simulink model "MZ_Simulink_AAI"  (R2020a)
settings: Solver=FixedStepAuto  StartTime=0.0  StopTime=10.0  FixedStep=1e-3  RelTol=1e-3  EnableMultiTasking=on
undefined symbols (not defined in the file or in its folder): D0, D1, D10, D11, D12, D13, D2, D3, D5, D6, D8, D9, Modes, PTA0, PTA1, PTA2, PTB9, PTC16, PTC17, PTC2, PTC4, PTD0, PTD1, PTD2, PTD3
libraries: frdmk64flib x12, simulink x1
settings Model: ExtModeTrigDuration=5  Creator=USER  LastModifiedBy=micha
settings OptimizationCC: EnhancedBackFolding=on  PassReuseOutputArgsAs=Individual arguments  ZeroExternalMemoryAtStartup=off  ZeroInternalMemoryAtStartup=off  MaxStackSize=64  OptimizeBlockOrder=speed  DifferentSizesBufferReuse=on  OptimizationCustomize=off  EfficientTunableParamExpr=on
settings DebuggingCC: ParameterTunabilityLossMsg=error
settings HardwareCC: ProdBitPerPointer=32  ProdBitPerSizeT=32  ProdBitPerPtrDiffT=32  ProdLargestAtomicInteger=Long  ProdLargestAtomicFloat=Double  ProdWordSize=32  ProdHWDeviceType=ARM Compatible->ARM Cortex
settings SFSimCC: MATLABDynamicMemAlloc=off
settings RTWCC: SystemTargetFile=ert.tlc  HardwareBoard=NXP FRDM-K64F  TemplateMakefile=ert_default_tmf  Toolchain=GNU Tools for ARM Embedded Processors
settings CodeAppCC: ForceParamTrailComments=on  IgnoreCustomStorageClasses=off  OperatorAnnotations=on  SimulinkDataObjDesc=on  SFDataObjDesc=on  InsertBlockDesc=on

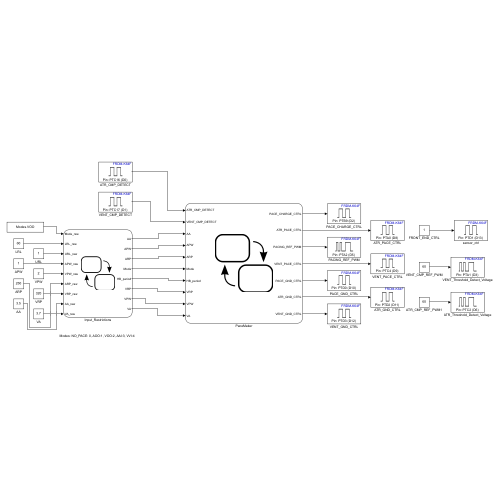
[thumbnail: Simulink's stored preview of the top-level diagram]
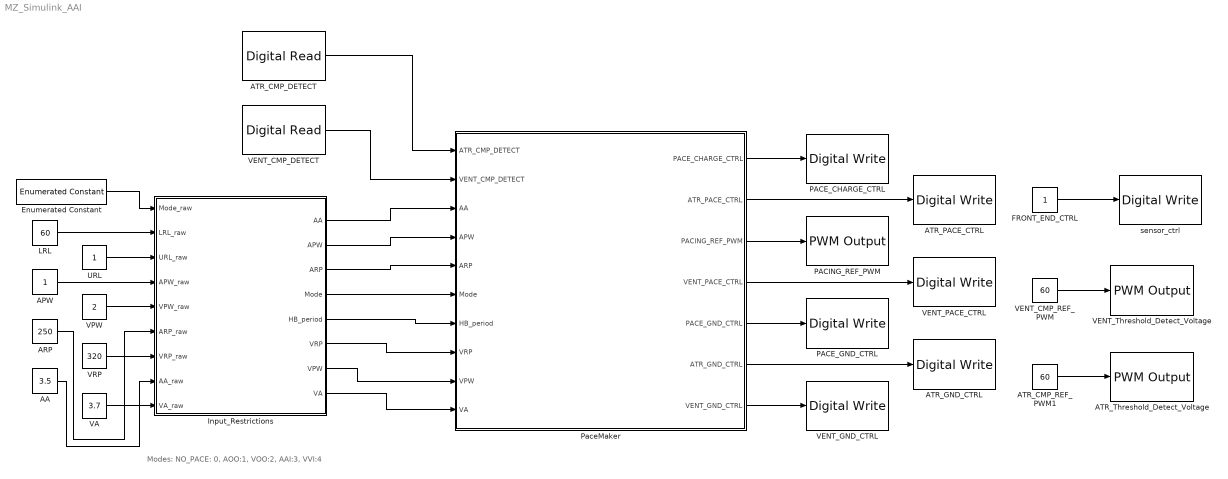
== system MZ_Simulink_AAI ==
  note: Modes: NO_PACE: 0, AOO:1, VOO:2, AAI:3, VVI:4
  AA : Constant  Value=3.5  OutDataTypeStr=single
  APW : Constant  OutDataTypeStr=uint8
  ARP : Constant  Value=250  OutDataTypeStr=uint16
  ATR_CMP_DETECT : frdmk64flib/Digital Read  Whichpin=PTC16 (D0)  SampleTime=-1
  ATR_CMP_REF_PWM1 : Constant  Value=60  OutDataTypeStr=uint8
  ATR_GND_CTRL : frdmk64flib/Digital Write  Whichpin=PTD2 (D11)
  ATR_PACE_CTRL : frdmk64flib/Digital Write  Whichpin=PTA0 (D8)
  ATR_Threshold_Detect_Voltage : frdmk64flib/PWM Output  Whichpin=PTC2 (D6)  InitialFrequency=2000  InitialDutyCycle=0
  Enumerated Constant : simulink/Sources/Enumerated Constant  OutDataTypeStr=Enum: Modes  Value=Modes.VOO  SampleTime=inf
  FRONT_END_CTRL : Constant
  Input_Restrictions : Stateflow chart  TreatAsAtomicUnit=on
      settings: PortSchema="{\"entries\":[{\"content\":{\"sides\":[{\"content\":{\"connectorIds\":[\"In1\",\"In2\",\"In3\",\"In4\",\"In5\",\"In6\",\"In7\",\"In8\",\"In9\"]},\"type\":\"ConnectorPlacement.EquallySpacedRectSide\",\"uuid\":\"6ca4b211-7758-4da9-b575-bca72ef3bde0\"},{\"content\":{\"connectorIds\":[\"Out6\",\"Out2\",\"Out4\",\"Out1\",\"Out8\",\"Out5\",\"Out3\",\"Out7\"],\"side\":\"RIGHT\"},\"type\":\"ConnectorPlacement.EquallySpacedRectSide\",\"uuid\":\"378f9a2c-b26e-4d35-a148-104ac3e5eb3b\"},{\"content\":{\"connectorIds\":[],\"side\":\"TOP\"},\"type\":\"ConnectorPlacement.EquallySpacedRectSide\",\"uuid\":\"60b5eb54-812a-46fe-8169-2e41f06633e9\"}]},\"type\":\"ConnectorPlacement.EquallySpacedConnector\",\"uuid\":\"c7c5acee-7732-4c88-8beb-9d710d5b10aa\"}],\"packageUris\":[\"http://schema.mathworks.com/mf0/Connector/R2020b\"],\"version\":\"1.0\"}"
  LRL : Constant  Value=60  OutDataTypeStr=uint8
  PACE_CHARGE_CTRL : frdmk64flib/Digital Write  Whichpin=PTB9 (D2)
  PACE_GND_CTRL : frdmk64flib/Digital Write  Whichpin=PTD0 (D10)
  PACING_REF_PWM : frdmk64flib/PWM Output  Whichpin=PTA2 (D5)  InitialFrequency=2000  InitialDutyCycle=0
  PaceMaker : Stateflow chart  TreatAsAtomicUnit=on
      settings: PortSchema="{\"entries\":[{\"content\":{\"sides\":[{\"content\":{\"connectorIds\":[\"In2\",\"In3\",\"In6\",\"In8\",\"In4\",\"In1\",\"In10\",\"In5\",\"In9\",\"In7\"]},\"type\":\"ConnectorPlacement.EquallySpacedRectSide\",\"uuid\":\"be11ab42-f218-4533-b046-48d6c6672980\"},{\"content\":{\"connectorIds\":[\"Out1\",\"Out2\",\"Out3\",\"Out4\",\"Out5\",\"Out6\",\"Out7\"],\"side\":\"RIGHT\"},\"type\":\"ConnectorPlacement.EquallySpacedRectSide\",\"uuid\":\"3184d97a-d95e-4f92-be49-d512e0e8be59\"},{\"content\":{\"connectorIds\":[],\"side\":\"TOP\"},\"type\":\"ConnectorPlacement.EquallySpacedRectSide\",\"uuid\":\"82a667a0-8f6e-4fe8-9d7d-d285af85bcaa\"}]},\"type\":\"ConnectorPlacement.EquallySpacedConnector\",\"uuid\":\"8df3a08e-b350-4a50-854d-64d5d1a667ae\"}],\"packageUris\":[\"http://schema.mathworks.com/mf0/Connector/R2020b\"],\"version\":\"1.0\"}"
  URL : Constant  OutDataTypeStr=uint8
  VA : Constant  Value=3.7  OutDataTypeStr=single
  VENT_CMP_DETECT : frdmk64flib/Digital Read  Whichpin=PTC17 (D1)  SampleTime=-1
  VENT_CMP_REF_PWM : Constant  Value=60  OutDataTypeStr=uint8
  VENT_GND_CTRL : frdmk64flib/Digital Write  Whichpin=PTD3 (D12)
  VENT_PACE_CTRL : frdmk64flib/Digital Write  Whichpin=PTC4 (D9)
  VENT_Threshold_Detect_Voltage : frdmk64flib/PWM Output  Whichpin=PTA1 (D3)  InitialFrequency=2000  InitialDutyCycle=0
  VPW : Constant  Value=2  OutDataTypeStr=uint8
  VRP : Constant  Value=320  OutDataTypeStr=uint16
  sensor_ctrl : frdmk64flib/Digital Write  Whichpin=PTD1 (D13)
  wires:
  VRP/1 -> Input_Restrictions/7(VRP_raw)
  URL/1 -> Input_Restrictions/3(URL_raw)
  Input_Restrictions/1(Mode) -> PaceMaker/1(Mode)
  APW/1 -> Input_Restrictions/4(APW_raw)
  VA/1 -> Input_Restrictions/9(VA_raw)
  AA/1 -> Input_Restrictions/8(AA_raw)
  Enumerated Constant/1 -> Input_Restrictions/1(Mode_raw)
  ARP/1 -> Input_Restrictions/6(ARP_raw)
  LRL/1 -> Input_Restrictions/2(LRL_raw)
  VPW/1 -> Input_Restrictions/5(VPW_raw)
  Input_Restrictions/4(ARP) -> PaceMaker/4(ARP)
  Input_Restrictions/5(VRP) -> PaceMaker/5(VRP)
  ATR_CMP_DETECT/1 -> PaceMaker/2(ATR_CMP_DETECT)
  VENT_CMP_DETECT/1 -> PaceMaker/3(VENT_CMP_DETECT)
  PaceMaker/1(PACE_CHARGE_CTRL) -> PACE_CHARGE_CTRL/1
  PaceMaker/2(ATR_PACE_CTRL) -> ATR_PACE_CTRL/1
  PaceMaker/3(PACING_REF_PWM) -> PACING_REF_PWM/1
  PaceMaker/4(VENT_PACE_CTRL) -> VENT_PACE_CTRL/1
  PaceMaker/5(PACE_GND_CTRL) -> PACE_GND_CTRL/1
  PaceMaker/6(ATR_GND_CTRL) -> ATR_GND_CTRL/1
  PaceMaker/7(VENT_GND_CTRL) -> VENT_GND_CTRL/1
  Input_Restrictions/6(AA) -> PaceMaker/6(AA)
  Input_Restrictions/7(VA) -> PaceMaker/7(VA)
  Input_Restrictions/2(APW) -> PaceMaker/8(APW)
  Input_Restrictions/3(VPW) -> PaceMaker/9(VPW)
  VENT_CMP_REF_PWM/1 -> VENT_Threshold_Detect_Voltage/1
  FRONT_END_CTRL/1 -> sensor_ctrl/1
  ATR_CMP_REF_PWM1/1 -> ATR_Threshold_Detect_Voltage/1
  Input_Restrictions/8(HB_period) -> PaceMaker/10(HB_period)

== stateflow chart MZ_Simulink_AAI/PaceMaker ==
  state AOO
    state Pace_ATR
      state Charge_PaceC_Discharge_BlockingC
        ATR_PACE_CTRL = false;
        VENT_PACE_CTRL = false;
        PACING_REF_PWM = cast(AA*100/5,'uint8');
        PACE_CHARGE_CTRL = true;
        PACE_GND_CTRL = true;
        VENT_GND_CTRL = false;
        ATR_GND_CTRL = true;
        inPace = false;
      state ATR_Pacing
        PACE_CHARGE_CTRL = false;
        PACE_GND_CTRL = true;
        VENT_PACE_CTRL = false;
        VENT_GND_CTRL = false;
        ATR_GND_CTRL = false;
        ATR_PACE_CTRL = true;
      (default) -> Charge_PaceC_Discharge_BlockingC
      AOO.Pace_ATR.ATR_Pacing -> Charge_PaceC_Discharge_BlockingC : after(APW,msec)
      Charge_PaceC_Discharge_BlockingC -> AOO.Pace_ATR.ATR_Pacing : after(HB_period-cast(APW,'single'),msec){inPace = true}
    (default) -> Pace_ATR
  state No_Pace
    PACE_CHARGE_CTRL = false;
    ATR_PACE_CTRL = false;
    PACING_REF_PWM = 0;
    VENT_PACE_CTRL = false;
    PACE_GND_CTRL = true;
    ATR_GND_CTRL = true;
    VENT_GND_CTRL = true;
    inPace = false;
  state VOO
    state Pace_VENT
      state Charge_PaceC_Discharge_Discharge_BlockingC
        ATR_PACE_CTRL = false;
        VENT_PACE_CTRL = false;
        PACING_REF_PWM = cast(VA*100/5,'uint8');
        PACE_CHARGE_CTRL = true;
        PACE_GND_CTRL = true;
        VENT_GND_CTRL = true;
        inPace = false;
      state VENT_Pacing
        PACE_CHARGE_CTRL=false;
        PACE_GND_CTRL=true;
        ATR_PACE_CTRL=false;
        ATR_GND_CTRL=false;
        VENT_GND_CTRL=false;
        VENT_PACE_CTRL=true;
      (default) -> Charge_PaceC_Discharge_Discharge_BlockingC
      VOO.Pace_VENT.VENT_Pacing -> Charge_PaceC_Discharge_Discharge_BlockingC : after(VPW,msec)
      Charge_PaceC_Discharge_Discharge_BlockingC -> VOO.Pace_VENT.VENT_Pacing : after(HB_period-cast(VPW,'single'),msec){inPace = true}
    (default) -> Pace_VENT
  state VVI
    state Sense
      ATR_PACE_CTRL = false;
      VENT_PACE_CTRL = false;
      PACING_REF_PWM = cast(VA*100/5,'uint8');
      PACE_CHARGE_CTRL = true;
    state VENT_Pacing
      PACE_CHARGE_CTRL=false;
      PACE_GND_CTRL=true;
      ATR_PACE_CTRL=false;
      ATR_GND_CTRL=false;
      VENT_GND_CTRL=false;
      VENT_PACE_CTRL=true;
    state wait
      PACE_GND_CTRL = true;
      VENT_PACE_CTRL = false;
      ATR_PACE_CTRL = false;
      ATR_GND_CTRL = false;
      VENT_GND_CTRL = true;
      inPace = false;
    (default) -> VVI.Sense
    VVI.Sense -> VVI.wait [order 1] : [VENT_CMP_DETECT == true]{waitInt = VRP;}
    VVI.Sense -> VVI.VENT_Pacing [order 2] : after(HB_period - cast(VRP,'single'),msec){waitInt = VRP - VPW; inPace = true;}
    VVI.wait -> VVI.Sense : after(waitInt,msec)
    VVI.VENT_Pacing -> VVI.wait : after(VPW,msec)
  state AAI
    state Sense
      ATR_PACE_CTRL = false;
      VENT_PACE_CTRL = false;
      PACING_REF_PWM = cast(AA*100/5,'uint8');
      PACE_CHARGE_CTRL = true;
    state ATR_Pacing
      PACE_CHARGE_CTRL = false;
      PACE_GND_CTRL = true;
      VENT_PACE_CTRL = false;
      VENT_GND_CTRL = false;
      ATR_GND_CTRL = false;
      ATR_PACE_CTRL = true;
    state wait
      PACE_GND_CTRL = true;
      VENT_PACE_CTRL = false;
      ATR_PACE_CTRL = false;
      VENT_GND_CTRL = false;
      ATR_GND_CTRL = true;
      inPace = false;
    (default) -> AAI.Sense
    AAI.Sense -> AAI.wait [order 1] : [ATR_CMP_DETECT == true]{waitInt = ARP;}
    AAI.Sense -> AAI.ATR_Pacing [order 2] : after(HB_period - cast(ARP,'single'),msec){waitInt = ARP - APW; inPace = true;}
    AAI.wait -> AAI.Sense : after(waitInt,msec)
    AAI.ATR_Pacing -> AAI.wait : after(APW,msec)
  (junction 22) -> AOO [order 2] : [Mode == Modes.AOO]
  AOO -> (junction 22) : [Mode ~=Modes.AOO && inPace == false]
  (default) -> No_Pace
  No_Pace -> (junction 22) : [Mode ~= Modes.NO_PACE]
  VOO -> (junction 22) : [Mode ~= Modes.VOO  && inPace == false]
  (junction 22) -> No_Pace [order 1] : [Mode == Modes.NO_PACE]
  (junction 22) -> VOO [order 3] : [Mode == Modes.VOO]
  (junction 22) -> VVI [order 4] : [Mode == Modes.VVI]
  (junction 22) -> AAI [order 5] : [Mode == Modes.AAI]
  AAI -> (junction 22) : [Mode ~= Modes.AAI  && inPace == false]
  VVI -> (junction 22) : [Mode ~= Modes.VVI  && inPace == false]
  data: Mode input Enum: Modes; ATR_CMP_DETECT input boolean; VENT_CMP_DETECT input boolean; ARP input uint16; VRP input uint16; AA input single; VA input single; APW input uint8; VPW input uint8; PACE_CHARGE_CTRL output boolean; ATR_PACE_CTRL output boolean; PACING_REF_PWM output uint8; VENT_PACE_CTRL output boolean; PACE_GND_CTRL output boolean; ATR_GND_CTRL output boolean; VENT_GND_CTRL output boolean; HB_period input single; inPace local boolean

== stateflow chart MZ_Simulink_AAI/Input_Restrictions ==
  state Restrictions
    Mode = Mode_raw;
    LRL = LRL_raw;
    URL = URL_raw;
    APW = APW_raw;
    VPW = VPW_raw;
    ARP = ARP_raw;
    VRP = VRP_raw;
    AA = AA_raw;
    VA = VA_raw;
    HB_period = 1000/(cast(LRL,'single')/60);
  (default) -> Restrictions
  data: Mode_raw input Enum: Modes; LRL_raw input uint8; URL_raw input uint8; APW_raw input uint8; VPW_raw input uint8; ARP_raw input uint16; VRP_raw input uint16; AA_raw input single; VA_raw input single; Mode output Enum: Modes; APW output uint8; VPW output uint8; ARP output uint16; VRP output uint16; AA output single; VA output single; LRL local uint8; URL local uint8; HB_period output single
